simulink model "simula_ajuste_mimo"  (R2018a)
settings: Solver=VariableStepAuto  StartTime=0.0  StopTime=Tsim  FixedStep=0.00001  RelTol=1e-3
undefined symbols (not defined in the file): delta, Ke, Kf, Kr, Ts, Tsim
libraries: cstblocks x5, simulink x1
settings Model: Creator=aluno-4  LastModifiedBy=marcus

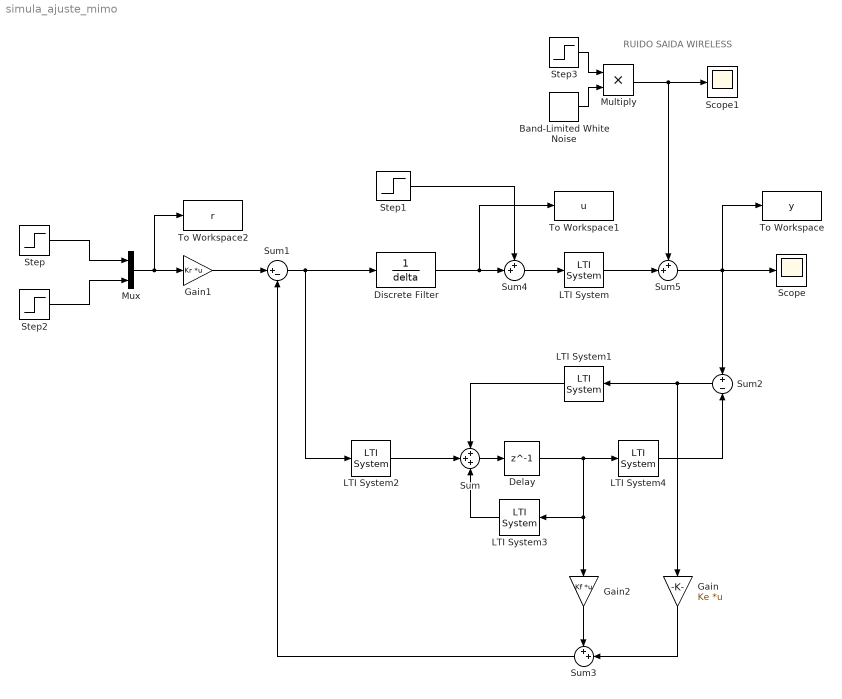
== system simula_ajuste_mimo ==
  note: RUIDO SAIDA WIRELESS
  Band-Limited White Noise : simulink/Sources/Band-Limited White Noise  Cov=Ts/5000  Ts=Ts/10  seed=[23341]
  Delay : Delay  DelayLength=1  SampleTime=Ts
  Discrete Filter : DiscreteFilter  Numerator=1  Denominator=delta  SampleTime=Ts
  Gain : Gain  Gain=Ke  Multiplication=Matrix(K*u)
  Gain1 : Gain  Gain=Kr  Multiplication=Matrix(K*u)
  Gain2 : Gain  Gain=Kf  Multiplication=Matrix(K*u)
  LTI System : cstblocks/LTI System  sys=P  IC=[]
  LTI System1 : cstblocks/LTI System  sys=D  IC=[]
  LTI System2 : cstblocks/LTI System  sys=B  IC=[]
  LTI System3 : cstblocks/LTI System  sys=A  IC=[]
  LTI System4 : cstblocks/LTI System  sys=H  IC=[]
  Multiply : Product
  Mux : Mux  Inputs=2
  Scope : Scope
  Scope1 : Scope
  Step : Step  Time=45*Tsim/100  Before=0.5  After=0.4  SampleTime=0
  Step1 : Step  Time=Tsim/2  After=0.5  SampleTime=0
  Step2 : Step  Time=0  After=0.3  SampleTime=0
  Step3 : Step  Time=4*Tsim/5  SampleTime=0
  Sum : Sum  Inputs=+++
  Sum1 : Sum  Inputs=|+-
  Sum2 : Sum  Inputs=+-
  Sum3 : Sum  Inputs=++|
  Sum4 : Sum  Inputs=++|
  Sum5 : Sum  Inputs=++|
  To Workspace : ToWorkspace  VariableName=y  SaveFormat=Timeseries  SampleTime=-1
  To Workspace1 : ToWorkspace  VariableName=u  SaveFormat=Timeseries  SampleTime=Ts
  To Workspace2 : ToWorkspace  VariableName=r  SaveFormat=Timeseries  SampleTime=-1
  wires:
  Sum3/1 -> Sum1/2
  Gain2/1 -> Sum3/1
  Step/1 -> Mux/1
  Sum1/1 -> LTI System2/1, Discrete Filter/1
  Sum4/1 -> LTI System/1
  Gain/1 -> Sum3/2
  Step2/1 -> Mux/2
  Discrete Filter/1 -> To Workspace1/1, Sum4/2
  LTI System2/1 -> Sum/2
  LTI System4/1 -> Sum2/2
  Sum2/1 -> LTI System1/1, Gain/1
  LTI System1/1 -> Sum/1
  Sum/1 -> Delay/1
  Mux/1 -> To Workspace2/1, Gain1/1
  Delay/1 -> LTI System4/1, Gain2/1, LTI System3/1
  LTI System3/1 -> Sum/3
  Step1/1 -> Sum4/1
  LTI System/1 -> Sum5/2
  Band-Limited White Noise/1 -> Multiply/2
  Step3/1 -> Multiply/1
  Multiply/1 -> Sum5/1, Scope1/1
  Gain1/1 -> Sum1/1
  Sum5/1 -> Sum2/1, To Workspace/1, Scope/1
